simulink model "kontrol_nelin_dec_zanem"  (R2020a)
settings: Solver=ode4  StartTime=0.0  StopTime=tfin  FixedStep=1  RelTol=1e-3  EnableMultiTasking=on
values from neighbouring files (symbols this model uses):
  Ca = 1e-6    (= 1e-06)    [dec_stat_dek.m]    (also in dec_w0_dek.m; dec_zanemarivanje.m; hinf.m; inverzija_potpuna.m)
  Cb = 1e-6    (= 1e-06)    [dec_stat_dek.m]    (also in dec_w0_dek.m; dec_zanemarivanje.m; hinf.m; inverzija_potpuna.m)
  Fae = 1/60    (= 0.0166666666667)    [dec_stat_dek.m]    (also in dec_w0_dek.m; dec_zanemarivanje.m; hinf.m; inverzija_potpuna.m)
  Fbe = 2/60    (= 0.0333333333333)    [dec_stat_dek.m]    (also in dec_w0_dek.m; dec_zanemarivanje.m; hinf.m; inverzija_potpuna.m)
  kv = 0.01    [dec_stat_dek.m]    (also in dec_w0_dek.m; dec_zanemarivanje.m; hinf.m; inverzija_potpuna.m)
  kw = 1e-14    [dec_stat_dek.m]    (also in dec_w0_dek.m; dec_zanemarivanje.m; hinf.m; inverzija_potpuna.m)
  pHe = -log10(H_plus_e)    [dec_stat_dek.m]    (also in dec_w0_dek.m; dec_zanemarivanje.m; hinf.m; inverzija_potpuna.m)
  pHstep = 0.0596    [kontrola_nelin_dec_zan_matlab.m]    (also in kontrola_nelin_svi_matlab.m = 5.96e-05)
  tu1_step1 = 1000    [kontrola_nelin_dec_zan_matlab.m]    (also in kontrola_nelin_svi_matlab.m)
  tu1_step2 = 3000    [kontrola_nelin_dec_zan_matlab.m]    (also in kontrola_nelin_svi_matlab.m = 10000)
  tu2_step1 = 5000    [kontrola_nelin_dec_zan_matlab.m]    (also in kontrola_nelin_svi_matlab.m = 1000)
  tu2_step2 = 7000    [kontrola_nelin_dec_zan_matlab.m]    (also in kontrola_nelin_svi_matlab.m = 10000)
  V = 30    [dec_stat_dek.m]    (also in dec_w0_dek.m; dec_zanemarivanje.m; hinf.m; inverzija_potpuna.m)
  xa0 = xae    (= 3.33333333333e-07)    [kontrola_nelin_dec_zan_matlab.m]    (also in kontrola_nelin_svi_matlab.m)
  xae = Fae*Ca/(Fae+Fbe)    (= 3.33333333333e-07)    [dec_stat_dek.m]    (also in dec_w0_dek.m; dec_zanemarivanje.m; hinf.m; inverzija_potpuna.m)
  xastep = 2.0819e-08    [kontrola_nelin_dec_zan_matlab.m]    (also in kontrola_nelin_svi_matlab.m = 2.274336e-08)
  xb0 = xbe    (= 5.55555555556e-07)    [kontrola_nelin_dec_zan_matlab.m]    (also in kontrola_nelin_svi_matlab.m)
undefined symbols (not defined in the file or in its folder): magnitude
libraries: cstblocks x1
settings Model: Creator=Sanja  LastModifiedBy=anaMceranic
settings DataIOCC: LimitDataPoints=on  SaveFormat=Array  ReturnWorkspaceOutputs=off
settings OptimizationCC: LifeSpan=inf
settings DebuggingCC: UnderspecifiedInitializationDetection=Classic  MergeDetectMultiDrivingBlocksExec=none  SolverPrmCheckMsg=warning  SFUnexpectedBacktrackingDiag=warning  SFNoUnconditionalDefaultTransitionDiag=warning  SFExecutionAtInitializationDiag=none  ArithmeticOperatorsInVariantConditions=warning
settings HardwareCC: ProdBitPerPointer=32  ProdBitPerSizeT=32  ProdBitPerPtrDiffT=32  ProdLargestAtomicFloat=None  ProdIntDivRoundTo=Undefined  ProdEndianess=Unspecified  ProdWordSize=32  ProdHWDeviceType=32-bit Generic
settings ModelReferenceCC: PropagateSignalLabelsOutOfModel=off
settings SFSimCC: SimUseLocalCustomCode=off  CustomCodeUndefinedFunction=UseInterfaceOnly
settings RTWCC: RTWUseLocalCustomCode=off
settings CodeAppCC: StateflowObjectComments=on
settings GRTTargetCC: TargetLangStandard=C89/C90 (ANSI)
settings ConfigComp: CovMetricSettings=dw  CovHtmlReporting=on  CovSaveCumulativeToWorkspaceVar=on  CovSaveSingleToWorkspaceVar=on  CovExternalEMLEnable=off

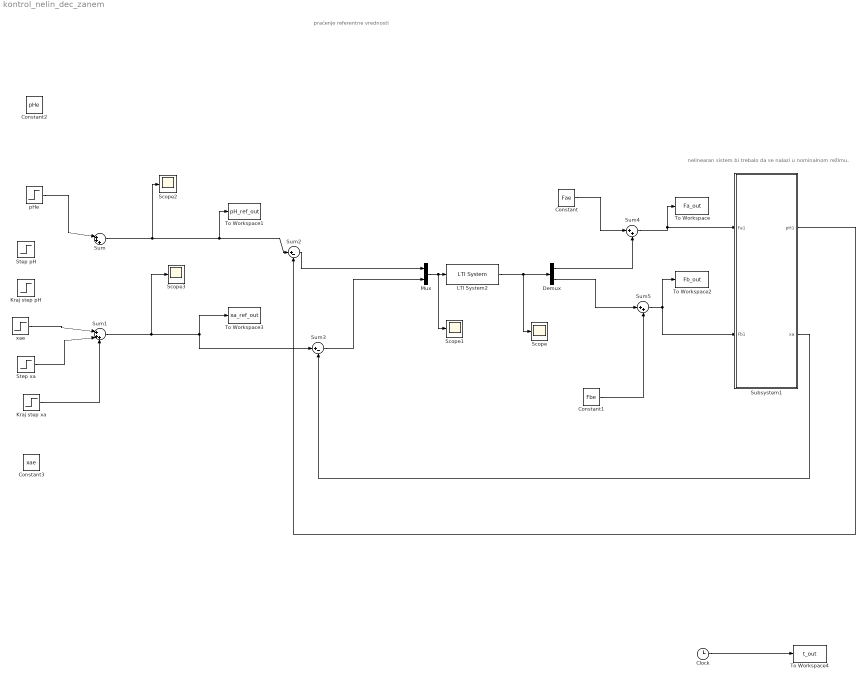
== system kontrol_nelin_dec_zanem ==
  note: praćenje referentne vrednosti
  note: nelinearan sistem bi trebalo da se nalazi u nominalnom režimu.
  Clock : Clock
  Constant : Constant  Value=Fae
  Constant1 : Constant  Value=Fbe
  Constant2 : Constant  Value=pHe
  Constant3 : Constant  Value=xae
  Demux : Demux  Outputs=2
  Kraj step pH : Step  Time=tu1_step2  After=-pHstep  SampleTime=0
  Kraj step xa : Step  Time=tu2_step2  After=-xastep  SampleTime=0
  LTI System2 : cstblocks/LTI System  sys=K_dec_z  IC=[]
  Mux : Mux  Inputs=2
  Scope{,1..3} (4 alike) : Scope
  Step pH : Step  Time=tu1_step1  After=pHstep  SampleTime=0
  Step xa : Step  Time=tu2_step1  After=xastep  SampleTime=0
  Subsystem1 : Subsystem
  Sum : Sum  Inputs=|+++
  Sum1 : Sum  Inputs=|+++
  Sum2 : Sum  Inputs=|+-
  Sum3 : Sum  Inputs=|+-
  Sum4 : Sum  Inputs=|++
  Sum5 : Sum  Inputs=|++
  To Workspace : ToWorkspace  VariableName=Fa_out  SampleTime=-1
  To Workspace1 : ToWorkspace  VariableName=pH_ref_out  SampleTime=-1
  To Workspace2 : ToWorkspace  VariableName=Fb_out  SampleTime=-1
  To Workspace3 : ToWorkspace  VariableName=xa_ref_out  SampleTime=-1
  To Workspace4 : ToWorkspace  VariableName=t_out  SampleTime=-1
  pHe : Step  Time=0  After=pHe  SampleTime=0
  xae : Step  Time=0  After=xae  SampleTime=0
  wires:
  Clock/1 -> To Workspace4/1
  Demux/1 -> Sum4/2
  Sum3/1 -> Mux/2
  Sum2/1 -> Mux/1
  Sum/1 -> Scope2/1, To Workspace1/1, Sum2/1
  Sum1/1 -> Scope3/1, To Workspace3/1, Sum3/1
  Subsystem1/1(pH1) -> Sum2/2
  Subsystem1/2(xa) -> Sum3/2
  Mux/1 -> Scope1/1, LTI System2/1
  LTI System2/1 -> Scope/1, Demux/1
  Sum4/1 -> Subsystem1/1(Fa1), To Workspace/1
  Constant/1 -> Sum4/1
  Demux/2 -> Sum5/1
  Constant1/1 -> Sum5/2
  Sum5/1 -> Subsystem1/2(Fb1), To Workspace2/1
  pHe/1 -> Sum/1
  xae/1 -> Sum1/1
  Step xa/1 -> Sum1/2
  Kraj step xa/1 -> Sum1/3

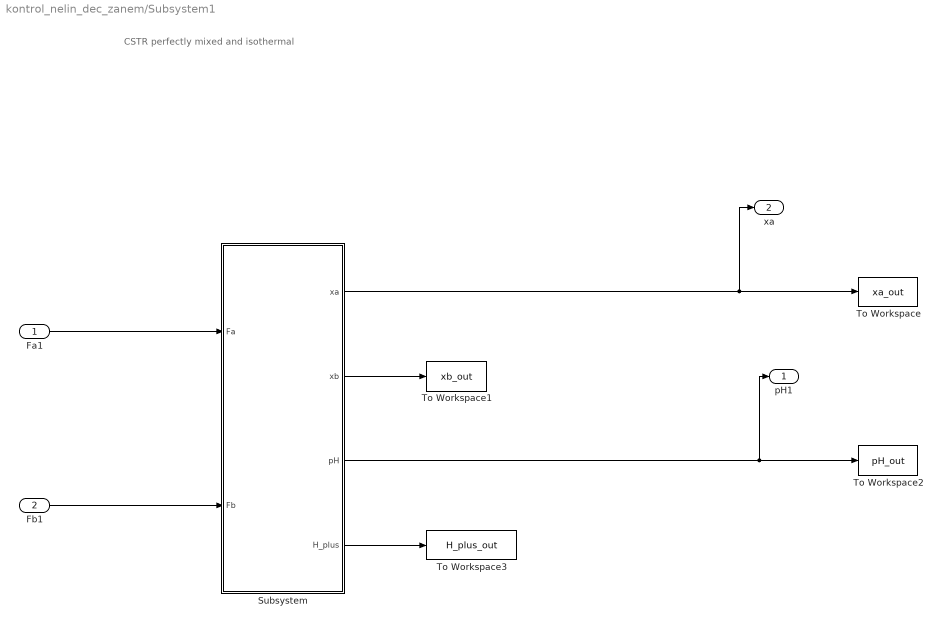
== system kontrol_nelin_dec_zanem/Subsystem1 ==
  note: CSTR perfectly mixed and isothermal
  Fa1 : Inport
  Fb1 : Inport  Port=2
  Subsystem : Subsystem
  To Workspace : ToWorkspace  VariableName=xa_out  SampleTime=-1
  To Workspace1 : ToWorkspace  VariableName=xb_out  SampleTime=-1
  To Workspace2 : ToWorkspace  VariableName=pH_out  SampleTime=-1
  To Workspace3 : ToWorkspace  VariableName=H_plus_out  SampleTime=-1
  pH1 : Outport
  xa : Outport  Port=2
  wires:
  Subsystem/2(xb) -> To Workspace1/1
  Subsystem/3(pH) -> pH1/1, To Workspace2/1
  Subsystem/4(H_plus) -> To Workspace3/1
  Subsystem/1(xa) -> xa/1, To Workspace/1
  Fb1/1 -> Subsystem/2(Fb)
  Fa1/1 -> Subsystem/1(Fa)

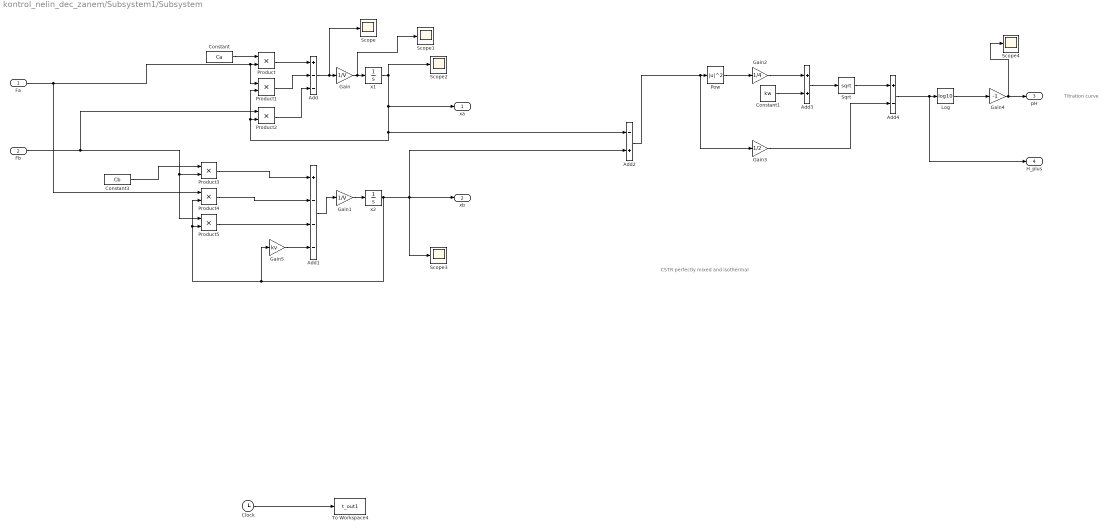
== system kontrol_nelin_dec_zanem/Subsystem1/Subsystem ==
  note: Titration curve
  note: CSTR perfectly mixed and isothermal
  Fa : Inport
  Fb : Inport  Port=2
  Add : Sum  Inputs=+--
  Add1 : Sum  Inputs=+---
  Add2 : Sum  Inputs=-+
  Add3 : Sum
  Add4 : Sum  Inputs=+-
  Clock : Clock
  Constant : Constant  Value=Ca
  Constant1 : Constant  Value=kw
  Constant3 : Constant  Value=Cb
  Gain : Gain  Gain=1/V
  Gain1 : Gain  Gain=1/V
  Gain2 : Gain  Gain=1/4
  Gain3 : Gain  Gain=1/2
  Gain4 : Gain  Gain=-1
  Gain5 : Gain  Gain=kv
  Log : Math  Operator=log10  SaturateOnIntegerOverflow=on
  Pow : Math  Operator=magnitude^2  SignedPower=on  RndMeth=Zero  SaturateOnIntegerOverflow=on
  Product{,1..5} (6 alike) : Product
  Scope{,1..4} (5 alike) : Scope
  Sqrt : Sqrt  SaturateOnIntegerOverflow=on
  To Workspace4 : ToWorkspace  VariableName=t_out1  SampleTime=-1
  x1 : Integrator  InitialCondition=xa0
  x2 : Integrator  InitialCondition=xb0
  xa : Outport
  xb : Outport  Port=2
  pH : Outport  Port=3
  H_plus : Outport  Port=4
  wires:
  Fb/1 -> Product5/1, Product3/2, Product2/1
  Constant3/1 -> Product3/1
  Product3/1 -> Add1/1
  Product5/1 -> Add1/3
  Product4/1 -> Add1/2
  x1/1 -> Scope2/1, Product1/2, Product2/2, Add2/1, xa/1
  Product2/1 -> Add/3
  x2/1 -> Add2/2, xb/1, Scope3/1, Gain5/1, Product4/2, Product5/2
  Add1/1 -> Gain1/1
  Gain1/1 -> x2/1
  Gain/1 -> Scope1/1, x1/1
  Fa/1 -> Product1/1, Product/2, Product4/1
  Product1/1 -> Add/2
  Product/1 -> Add/1
  Add/1 -> Scope/1, Gain/1
  Constant/1 -> Product/1
  Add2/1 -> Gain3/1, Pow/1
  Pow/1 -> Gain2/1
  Gain2/1 -> Add3/1
  Constant1/1 -> Add3/2
  Add3/1 -> Sqrt/1
  Sqrt/1 -> Add4/1
  Gain3/1 -> Add4/2
  Add4/1 -> H_plus/1, Log/1
  Log/1 -> Gain4/1
  Gain4/1 -> Scope4/1, pH/1
  Clock/1 -> To Workspace4/1
  Gain5/1 -> Add1/4
